simulink model "Altitude_SMCIBVS_RBFSMC"  (R2024b)
settings: Solver=FixedStepAuto  StartTime=0.0  StopTime=30  FixedStep=dT  RelTol=1e-3
InitFcn:
  | mass = 1; L = 0.2;
  | Ix = 0.008;
  | Iy = 0.008;
  | Iz = 0.017;
  | c = 0.088;
  | 
  | O = [0; 0; 0];        % world origin frame
  | C = [0; 0; 0.1];  % camera origin frame
  | 
  | d_initial = C - O;            % distance between camera and world frame
  | ang_initial = [0*pi/180  0*pi/180  0*pi/180];  % initial orientation, [pi 0 pi/2]
  | ang_final = [0*pi/180  0*pi/180  0*pi/180];
  | init_pose = [C ; ang_initial'];
  | d_final=[0; 0; 2];
  | dT=0.01;
  | g = 9.81;
  | %mass = 1; L = 0.6;
  | %Ix = 0.85;
  | %Iy = 0.85;
  | %c = 0.088;
  | 
  | p1 = [0.1; 0.1; 0.05];
  | p2 = [-0.1; 0.1; 0.05];
  | p3 = [0.1; -0.1; 0.05];
  | p4 = [-0.1; -0.1; 0.05];
  | % refcence
  | Rx = [1   0       0   ;
  |       0 cos(ang_final(1)) -sin(ang_final(1));
  |       0 sin(ang_final(1)) cos(ang_final(1))];
  | Ry = [cos(ang_final(2)) 0 sin(ang_final(2)) ;
  |        0     1   0    ;
  |      -sin(ang_final(2)) 0 cos(ang_final(2))];
  | 
  | Rz = [cos(ang_final(3)) -sin(ang_final(3)) 0;
  |       sin(ang_final(3))  cos(ang_final(3)) 0;
  |        0      0     1];
  | Rc = Rz * Ry * Rx;% body to inertial
  | Twc = [Rc            d_final;
  |       zeros(1,3)     1];
  | p_cam1 = Twc^-1 * [p1;1];   % point's position in camera frame
  | p_cam2 = Twc^-1 * [p2;1];
  | p_cam3 = Twc^-1 * [p3;1];   % point's position in camera frame
  | p_cam4 = Twc^-1 * [p4;1];
  | 
  | x_proj1 = p_cam1(1)/(p_cam1(3));%p_tilde1(1)/p_cam1(3);
  | y_proj1 = p_cam1(2)/(p_cam1(3));%p_tilde1(2)/p_cam1(3);
  | 
  | x_proj2 =p_cam2(1)/(p_cam2(3));% p_tilde2(1)/p_cam2(3);
  | y_proj2 =p_cam2(2)/(p_cam2(3));% p_tilde2(2)/p_cam2(3);
  | 
  | x_proj3 =p_cam3(1)/(p_cam3(3));% p_tilde1(1)/p_cam1(3);
  | y_proj3 =p_cam3(2)/(p_cam3(3));% p_tilde1(2)/p_cam1(3);
  | 
  | %
  | x_proj4 =p_cam4(1)/(p_cam4(3));% p_tilde2(1)/p_cam2(3);
  | y_proj4 =p_cam4(2)/(p_cam4(3));% p_tilde2(2)/p_cam2(3);
  | 
  | %%
  | ref1 = [x_proj1; y_proj1];
  | ref2 = [x_proj2; y_proj2];
  | ref3 = [x_proj3; y_proj3];
  | ref4 = [x_proj4; y_proj4];
  | 
  | ref = [ref1; ref2;ref3; ref4];
  | % control
  | %%k=[3.1383    2.9662    0.5    1.3]; %for altitude
  | k=[9.6489 9.5949 8.4692 4.5873];%for altitude new
  | 
  | kp=[k(1) k(1) k(2) k(1) k(1) k(1)];
  | kd=[k(3) k(3) k(4) k(3) k(3) k(3)];
  | %k=[1.5129    2.6987    1.6430    0.0242];%for position
  | %kp=[k(1) k(1) 5.2 k(3) k(3) 2];
  | %kd=[k(2) k(2) 4.5 k(4) k(4) 2.5];
  | 
  | Kp = diag(kp);
  | Kd = diag(kd);
  | 
  | %Rx = [1   0       0   ;
  | %      0 cos(ang_initial(1)) -sin(ang_initial(1));
  | %      0 sin(ang_initial(1)) cos(ang_initial(1))];
  | %Ry = [cos(ang_initial(2)) 0 sin(ang_initial(2)) ;
  | %       0     1   0    ;
  | %     -sin(ang_initial(2)) 0 cos(ang_initial(2))];
  | 
  | %Rz = [cos(ang_initial(3)) -sin(ang_initial(3)) 0;
  | %      sin(ang_initial(3))  cos(ang_initial(3)) 0;
  | %       0      0     1];
  | %Rc = Rz * Ry * Rx;% body to inertial
  | %Twc = [Rc            d_initial;
  | %      zeros(1,3)     1];
  | %p_cam1 = Twc^-1 * [p1;1];   % point's position in camera frame
  | %p_cam2 = Twc^-1 * [p2;1];
  | %p_cam3 = Twc^-1 * [p3;1];
  | %p_cam4 = Twc^-1 * [p4;1];
  | 
  | %x_proj1 = p_cam1(1)/(p_cam1(3));%p_tilde1(1)/p_cam1(3);
  | %y_proj1 = p_cam1(2)/(p_cam1(3));%p_tilde1(2)/p_cam1(3);
  | %Zc1 = p_cam1(3);
  | %x_proj2 =p_cam2(1)/(p_cam2(3));% p_tilde2(1)/p_cam2(3);
  | %y_proj2 =p_cam2(2)/(p_cam2(3));% p_tilde2(2)/p_cam2(3);
  | %Zc2 = p_cam2(3);
  | %x_proj3 = p_cam3(1)/(p_cam3(3));%p_tilde1(1)/p_cam1(3);
  | %y_proj3 = p_cam3(2)/(p_cam3(3));%p_tilde1(2)/p_cam1(3);
  | %Zc3 = p_cam3(3);
  | %x_proj4 =p_cam4(1)/(p_cam4(3));% p_tilde2(1)/p_cam2(3);
  | %y_proj4 =p_cam4(2)/(p_cam4(3));% p_tilde2(2)/p_cam2(3);
  | %Zc4 = p_cam4(3);
  | 
  | %ini_projection  = [x_proj1; y_proj1; Zc1; x_proj2; y_proj2; Zc2;x_proj3; y_proj3; Zc3; x_proj4; y_proj4; Zc4];
libraries: arduino_io_lib x1
settings Model: Creator=k513  LastModifiedBy=mohsen
settings DataIOCC: ReturnWorkspaceOutputs=off
settings ModelReferenceCC: EnableRefExpFcnMdlSchedulingChecks=on
settings RTWCC: GPUComputeCapability=3.5

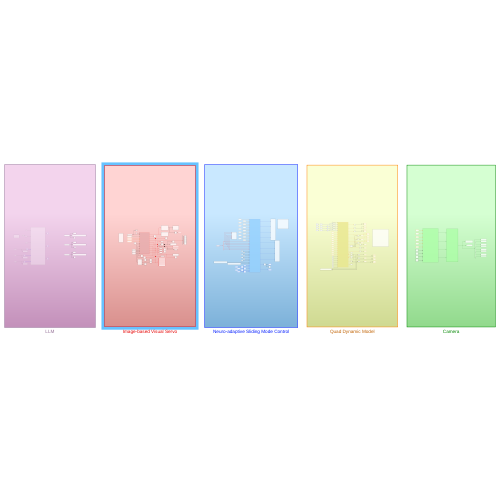
[thumbnail: Simulink's stored preview of the top-level diagram]
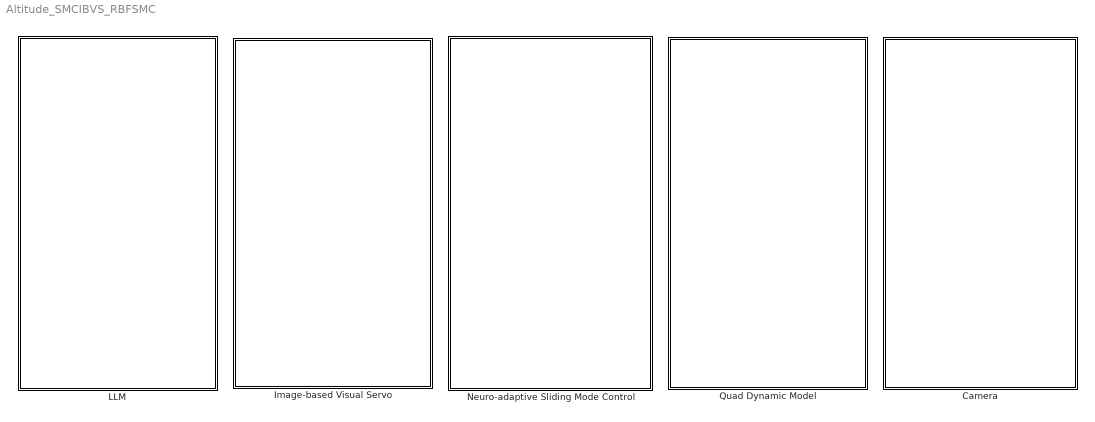
== system Altitude_SMCIBVS_RBFSMC ==
  Camera : Subsystem
  Image-based Visual Servo : Subsystem
  LLM : Subsystem
  Neuro-adaptive Sliding Mode Control : Subsystem
  Quad Dynamic Model : Subsystem

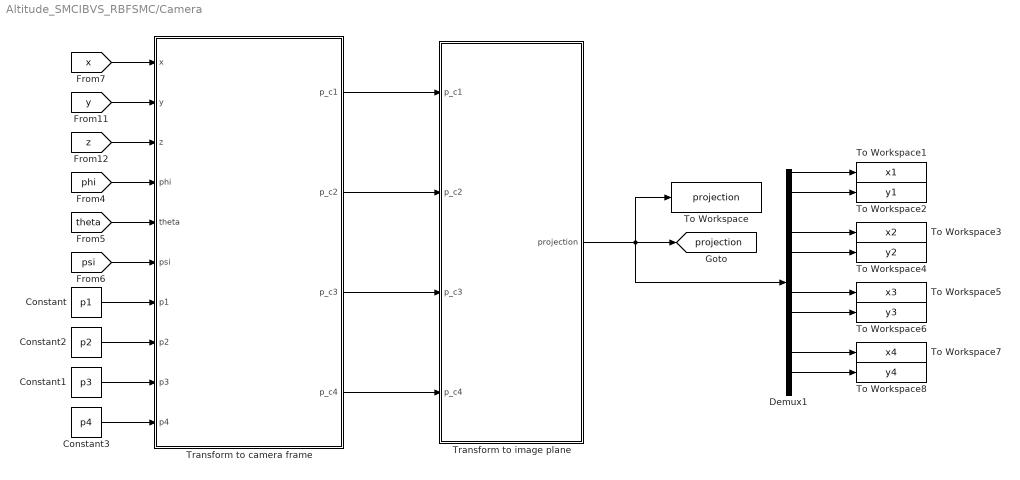
== system Altitude_SMCIBVS_RBFSMC/Camera ==
  Constant : Constant  Value=p1
  Constant1 : Constant  Value=p3
  Constant2 : Constant  Value=p2
  Constant3 : Constant  Value=p4
  Demux1 : Demux  Outputs=12
  To Workspace : ToWorkspace  VariableName=projection  SampleTime=-1
      settings: Save2DSignal=2-D array (concatenate along first dimension)
  To Workspace1 : ToWorkspace  VariableName=x1  SampleTime=-1
      settings: Save2DSignal=2-D array (concatenate along first dimension)
  To Workspace2 : ToWorkspace  VariableName=y1  SampleTime=-1
      settings: Save2DSignal=2-D array (concatenate along first dimension)
  To Workspace3 : ToWorkspace  VariableName=x2  SampleTime=-1
      settings: Save2DSignal=2-D array (concatenate along first dimension)
  To Workspace4 : ToWorkspace  VariableName=y2  SampleTime=-1
      settings: Save2DSignal=2-D array (concatenate along first dimension)
  To Workspace5 : ToWorkspace  VariableName=x3  SampleTime=-1
      settings: Save2DSignal=2-D array (concatenate along first dimension)
  To Workspace6 : ToWorkspace  VariableName=y3  SampleTime=-1
      settings: Save2DSignal=2-D array (concatenate along first dimension)
  To Workspace7 : ToWorkspace  VariableName=x4  SampleTime=-1
      settings: Save2DSignal=2-D array (concatenate along first dimension)
  To Workspace8 : ToWorkspace  VariableName=y4  SampleTime=-1
      settings: Save2DSignal=2-D array (concatenate along first dimension)
  Transform to camera frame : MATLAB Function  TreatAsAtomicUnit=on
  Transform to image plane : MATLAB Function  TreatAsAtomicUnit=on
  tag scope: projection=global
  wires:
  Transform to camera frame/1(p_c1) -> Transform to image plane/1(p_c1)
  Transform to camera frame/2(p_c2) -> Transform to image plane/2(p_c2)
  Transform to camera frame/3(p_c3) -> Transform to image plane/3(p_c3)
  Transform to camera frame/4(p_c4) -> Transform to image plane/4(p_c4)
  Demux1/2 -> To Workspace2/1
  Demux1/1 -> To Workspace1/1
  Transform to image plane/1(projection) -> To Workspace/1, Demux1/1, [projection]
  Demux1/11 -> To Workspace8/1
  Demux1/10 -> To Workspace7/1
  Demux1/8 -> To Workspace6/1
  Demux1/7 -> To Workspace5/1
  Demux1/5 -> To Workspace4/1
  Demux1/4 -> To Workspace3/1
  Constant/1 -> Transform to camera frame/7(p1)
  Constant2/1 -> Transform to camera frame/8(p2)
  Constant1/1 -> Transform to camera frame/9(p3)
  Constant3/1 -> Transform to camera frame/10(p4)
  [x] -> Transform to camera frame/1(x)
  [y] -> Transform to camera frame/2(y)
  [z] -> Transform to camera frame/3(z)
  [phi] -> Transform to camera frame/4(phi)
  [theta] -> Transform to camera frame/5(theta)
  [psi] -> Transform to camera frame/6(psi)

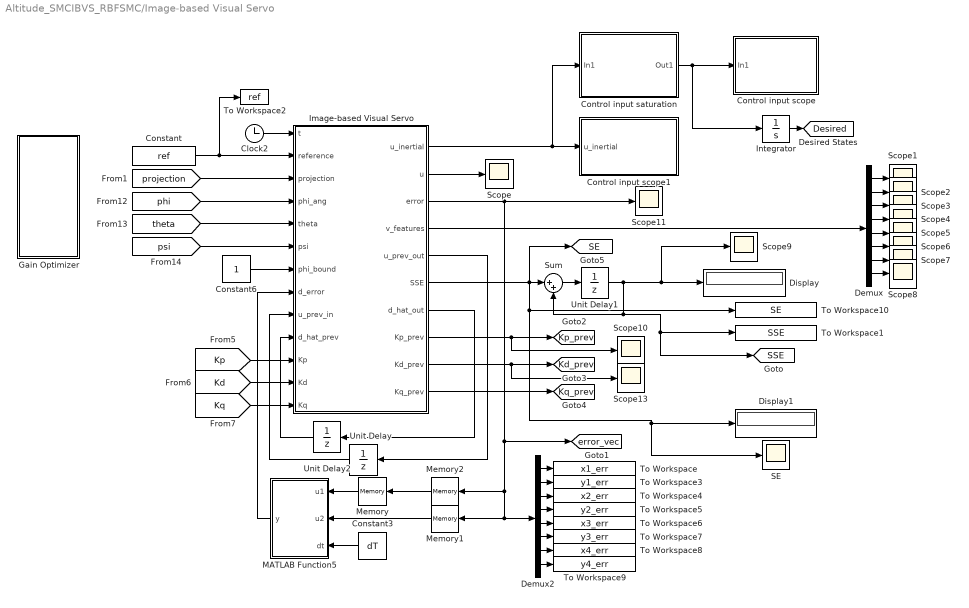
== system Altitude_SMCIBVS_RBFSMC/Image-based Visual Servo ==
  Clock2 : Clock
  Constant : Constant  Value=ref
  Constant3 : Constant  Value=dT
  Constant6 : Constant
  Control input saturation : Subsystem
  Control input scope : Subsystem
  Control input scope1 : Subsystem
  Demux : Demux  Outputs=8
  Demux2 : Demux  Outputs=8
  Display : Display
  Display1 : Display
  Gain Optimizer : Subsystem
  Image-based Visual Servo : MATLAB Function  TreatAsAtomicUnit=on
  Integrator : Integrator
  MATLAB Function5 : MATLAB Function  TreatAsAtomicUnit=on
  Memory : Memory  InitialCondition=zeros(8,1)
  Memory1 : Memory  InitialCondition=zeros(8,1)
  Memory2 : Memory  InitialCondition=zeros(8,1)
  SE : Scope
  Scope{,1..11,13} (13 alike) : Scope
  Sum : Sum  Inputs=|++
  To Workspace : ToWorkspace  VariableName=x1_err  SampleTime=-1
      settings: Save2DSignal=2-D array (concatenate along first dimension)
  To Workspace1 : ToWorkspace  VariableName=SSE  SampleTime=-1
      settings: Save2DSignal=2-D array (concatenate along first dimension)
  To Workspace10 : ToWorkspace  VariableName=SE  SampleTime=-1
      settings: Save2DSignal=2-D array (concatenate along first dimension)
  To Workspace2 : ToWorkspace  VariableName=ref  SampleTime=-1
      settings: Save2DSignal=2-D array (concatenate along first dimension)
  To Workspace3 : ToWorkspace  VariableName=y1_err  SampleTime=-1
      settings: Save2DSignal=2-D array (concatenate along first dimension)
  To Workspace4 : ToWorkspace  VariableName=x2_err  SampleTime=-1
      settings: Save2DSignal=2-D array (concatenate along first dimension)
  To Workspace5 : ToWorkspace  VariableName=y2_err  SampleTime=-1
      settings: Save2DSignal=2-D array (concatenate along first dimension)
  To Workspace6 : ToWorkspace  VariableName=x3_err  SampleTime=-1
      settings: Save2DSignal=2-D array (concatenate along first dimension)
  To Workspace7 : ToWorkspace  VariableName=y3_err  SampleTime=-1
      settings: Save2DSignal=2-D array (concatenate along first dimension)
  To Workspace8 : ToWorkspace  VariableName=x4_err  SampleTime=-1
      settings: Save2DSignal=2-D array (concatenate along first dimension)
  To Workspace9 : ToWorkspace  VariableName=y4_err  SampleTime=-1
      settings: Save2DSignal=2-D array (concatenate along first dimension)
  Unit Delay : UnitDelay  SampleTime=-1  HasFrameUpgradeWarning=on
  Unit Delay1 : UnitDelay  SampleTime=-1  HasFrameUpgradeWarning=on
  Unit Delay2 : UnitDelay  SampleTime=-1  HasFrameUpgradeWarning=on
  tag scope: Desired=global, Kd_prev=global, Kp_prev=global, Kq_prev=global, SE=global, SSE=global, error_vec=global
  wires:
  Memory/1 -> MATLAB Function5/1(u1)
  Constant/1 -> To Workspace2/1, Image-based Visual Servo/2(reference)
  [phi] -> Image-based Visual Servo/4(phi_ang)
  [theta] -> Image-based Visual Servo/5(theta)
  [psi] -> Image-based Visual Servo/6(psi)
  Image-based Visual Servo/3(error) -> Scope11/1, Demux2/1, Memory1/1, Memory2/1, [error_vec]
  [projection] -> Image-based Visual Servo/3(projection)
  Clock2/1 -> Image-based Visual Servo/1(t)
  Constant3/1 -> MATLAB Function5/3(dt)
  MATLAB Function5/1(y) -> Image-based Visual Servo/8(d_error)
  Memory1/1 -> MATLAB Function5/2(u2)
  Memory2/1 -> Memory/1
  Demux2/1 -> To Workspace/1
  Demux2/2 -> To Workspace3/1
  Demux2/3 -> To Workspace4/1
  Demux2/4 -> To Workspace5/1
  Demux2/5 -> To Workspace6/1
  Demux2/6 -> To Workspace7/1
  Demux2/7 -> To Workspace8/1
  Demux2/8 -> To Workspace9/1
  Integrator/1 -> [Desired]
  Control input saturation/1(Out1) -> Integrator/1, Control input scope/1(In1)
  Image-based Visual Servo/1(u_inertial) -> Control input saturation/1(In1), Control input scope1/1(u_inertial)
  Image-based Visual Servo/2(u) -> Scope/1
  Constant6/1 -> Image-based Visual Servo/7(phi_bound)
  Image-based Visual Servo/4(v_features) -> Demux/1
  Demux/1 -> Scope1/1
  Demux/2 -> Scope2/1
  Demux/3 -> Scope3/1
  Demux/4 -> Scope4/1
  Demux/5 -> Scope5/1
  Demux/6 -> Scope6/1
  Demux/7 -> Scope7/1
  Demux/8 -> Scope8/1
  Image-based Visual Servo/5(u_prev_out) -> Unit Delay/1
  Unit Delay/1 -> Image-based Visual Servo/9(u_prev_in)
  Image-based Visual Servo/6(SSE) -> To Workspace10/1, SE/1, Display1/1, Sum/1, [SE]
  Sum/1 -> Unit Delay1/1
  Unit Delay1/1 -> [SSE], To Workspace1/1, Sum/2, Scope9/1, Display/1
  Image-based Visual Servo/7(d_hat_out) -> Unit Delay2/1
  Unit Delay2/1 -> Image-based Visual Servo/10(d_hat_prev)
  Image-based Visual Servo/8(Kp_prev) -> Scope10/1, [Kp_prev]
  Image-based Visual Servo/9(Kd_prev) -> [Kd_prev], Scope13/1
  Image-based Visual Servo/10(Kq_prev) -> [Kq_prev]
  [Kp] -> Image-based Visual Servo/11(Kp)
  [Kd] -> Image-based Visual Servo/12(Kd)
  [Kq] -> Image-based Visual Servo/13(Kq)

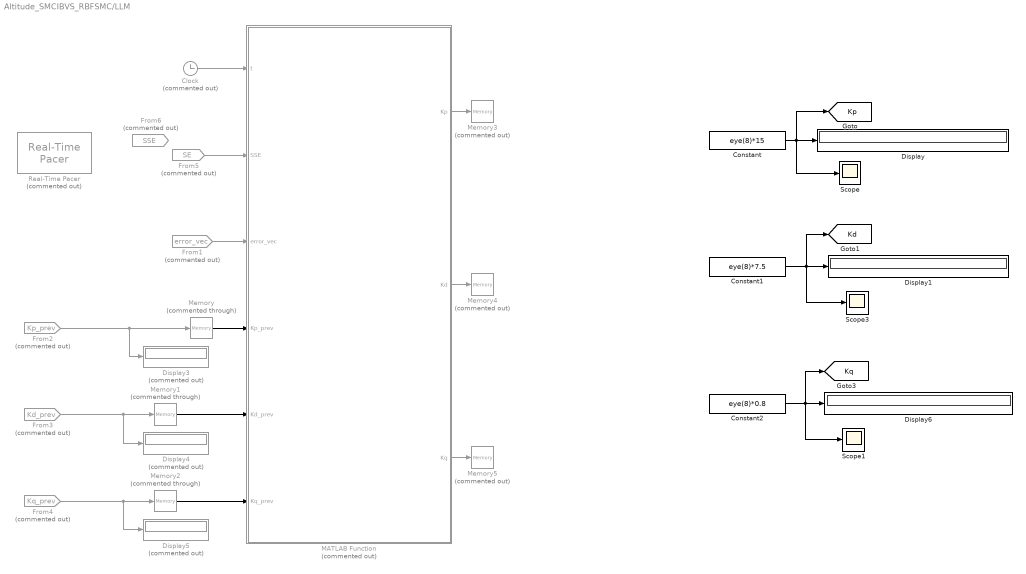
== system Altitude_SMCIBVS_RBFSMC/LLM ==
  Clock : Clock  Commented=on
  Constant : Constant  Value=eye(8)*15
  Constant1 : Constant  Value=eye(8)*7.5
  Constant2 : Constant  Value=eye(8)*0.8
  Display : Display
  Display1 : Display
  Display3 : Display  Commented=on
  Display4 : Display  Commented=on
  Display5 : Display  Commented=on
  Display6 : Display
  From1 : From  Commented=on  GotoTag=error_vec  TagVisibility=global
  From2 : From  Commented=on  GotoTag=Kp_prev  TagVisibility=global
  From3 : From  Commented=on  GotoTag=Kd_prev  TagVisibility=global
  From4 : From  Commented=on  GotoTag=Kq_prev  TagVisibility=global
  From5 : From  Commented=on  GotoTag=SE  TagVisibility=global
  From6 : From  Commented=on  GotoTag=SSE  TagVisibility=global
  MATLAB Function : MATLAB Function  Commented=on  TreatAsAtomicUnit=on
  Memory : Memory  Commented=through
  Memory1 : Memory  Commented=through
  Memory2 : Memory  Commented=through
  Memory3 : Memory  Commented=on
  Memory4 : Memory  Commented=on
  Memory5 : Memory  Commented=on
  Real-Time Pacer : arduino_io_lib/Real-Time Pacer  Commented=on  simTimePerRealTime=1
      settings: SourceProductName=Arduino IO Library
  Scope : Scope
  Scope1 : Scope
  Scope3 : Scope
  tag scope: Kd=global, Kp=global, Kq=global
  wires:
  MATLAB Function/1(Kp) -> Memory3/1
  MATLAB Function/3(Kq) -> Memory5/1
  MATLAB Function/2(Kd) -> Memory4/1
  Clock/1 -> MATLAB Function/1(t)
  From1/1 -> MATLAB Function/3(error_vec)
  From5/1 -> MATLAB Function/2(SSE)
  Memory/1 -> MATLAB Function/4(Kp_prev)
  Memory1/1 -> MATLAB Function/5(Kd_prev)
  Memory2/1 -> MATLAB Function/6(Kq_prev)
  From2/1 -> Display3/1, Memory/1
  From3/1 -> Display4/1, Memory1/1
  From4/1 -> Memory2/1, Display5/1
  Constant/1 -> Scope/1, [Kp], Display/1
  Constant1/1 -> Scope3/1, [Kd], Display1/1
  Constant2/1 -> Scope1/1, Display6/1, [Kq]

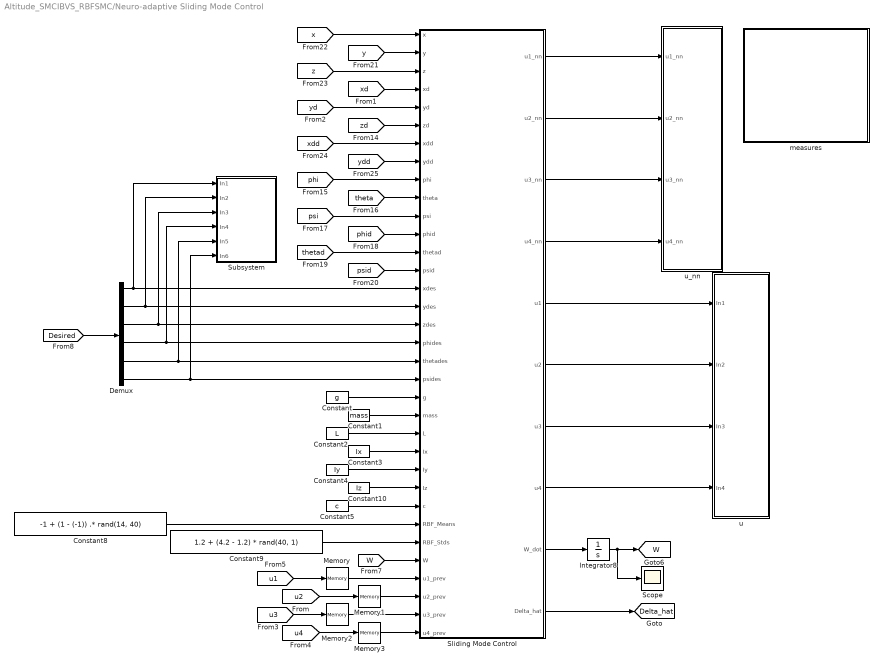
== system Altitude_SMCIBVS_RBFSMC/Neuro-adaptive Sliding Mode Control ==
  Constant : Constant  Value=g
  Constant1 : Constant  Value=mass
  Constant10 : Constant  Value=Iz
  Constant2 : Constant  Value=L
  Constant3 : Constant  Value=Ix
  Constant4 : Constant  Value=Iy
  Constant5 : Constant  Value=c
  Constant8 : Constant  Value=-1 + (1 - (-1)) .* rand(14, 40)
  Constant9 : Constant  Value=1.2 + (4.2 - 1.2) * rand(40, 1)
  Demux : Demux  Outputs=6
  Integrator8 : Integrator  InitialCondition=zeros(40, 4)
  Memory{,1..3} (4 alike) : Memory
  Scope : Scope
  Sliding Mode Control : MATLAB Function  TreatAsAtomicUnit=on
  Subsystem : Subsystem
  measures : Subsystem
  u : Subsystem
  u_nn : Subsystem
  tag scope: Delta_hat=global, W=global
  wires:
  [theta] -> Sliding Mode Control/10(theta)
  [zd] -> Sliding Mode Control/6(zd)
  [yd] -> Sliding Mode Control/5(yd)
  [xdd] -> Sliding Mode Control/7(xdd)
  [thetad] -> Sliding Mode Control/13(thetad)
  [phid] -> Sliding Mode Control/12(phid)
  [psi] -> Sliding Mode Control/11(psi)
  [ydd] -> Sliding Mode Control/8(ydd)
  [y] -> Sliding Mode Control/2(y)
  [phi] -> Sliding Mode Control/9(phi)
  [xd] -> Sliding Mode Control/4(xd)
  [psid] -> Sliding Mode Control/14(psid)
  [x] -> Sliding Mode Control/1(x)
  [z] -> Sliding Mode Control/3(z)
  [Desired] -> Demux/1
  Demux/3 -> Subsystem/3(In3), Sliding Mode Control/17(zdes)
  Constant/1 -> Sliding Mode Control/21(g)
  Constant1/1 -> Sliding Mode Control/22(mass)
  Constant2/1 -> Sliding Mode Control/23(L)
  Constant3/1 -> Sliding Mode Control/24(Ix)
  Constant4/1 -> Sliding Mode Control/25(Iy)
  Constant5/1 -> Sliding Mode Control/27(c)
  Constant10/1 -> Sliding Mode Control/26(Iz)
  Constant9/1 -> Sliding Mode Control/29(RBF_Stds)
  Constant8/1 -> Sliding Mode Control/28(RBF_Means)
  Sliding Mode Control/9(W_dot) -> Integrator8/1
  [u1] -> Memory/1
  [u2] -> Memory1/1
  [u3] -> Memory2/1
  [u4] -> Memory3/1
  Memory/1 -> Sliding Mode Control/31(u1_prev)
  Memory1/1 -> Sliding Mode Control/32(u2_prev)
  Memory2/1 -> Sliding Mode Control/33(u3_prev)
  Memory3/1 -> Sliding Mode Control/34(u4_prev)
  Sliding Mode Control/10(Delta_hat) -> [Delta_hat]
  Integrator8/1 -> Scope/1, [W]
  [W] -> Sliding Mode Control/30(W)
  Demux/1 -> Subsystem/1(In1), Sliding Mode Control/15(xdes)
  Demux/2 -> Subsystem/2(In2), Sliding Mode Control/16(ydes)
  Demux/4 -> Subsystem/4(In4), Sliding Mode Control/18(phides)
  Demux/5 -> Subsystem/5(In5), Sliding Mode Control/19(thetades)
  Demux/6 -> Subsystem/6(In6), Sliding Mode Control/20(psides)
  Sliding Mode Control/1(u1_nn) -> u_nn/1(u1_nn)
  Sliding Mode Control/2(u2_nn) -> u_nn/2(u2_nn)
  Sliding Mode Control/3(u3_nn) -> u_nn/3(u3_nn)
  Sliding Mode Control/4(u4_nn) -> u_nn/4(u4_nn)
  Sliding Mode Control/5(u1) -> u/1(In1)
  Sliding Mode Control/6(u2) -> u/2(In2)
  Sliding Mode Control/7(u3) -> u/3(In3)
  Sliding Mode Control/8(u4) -> u/4(In4)

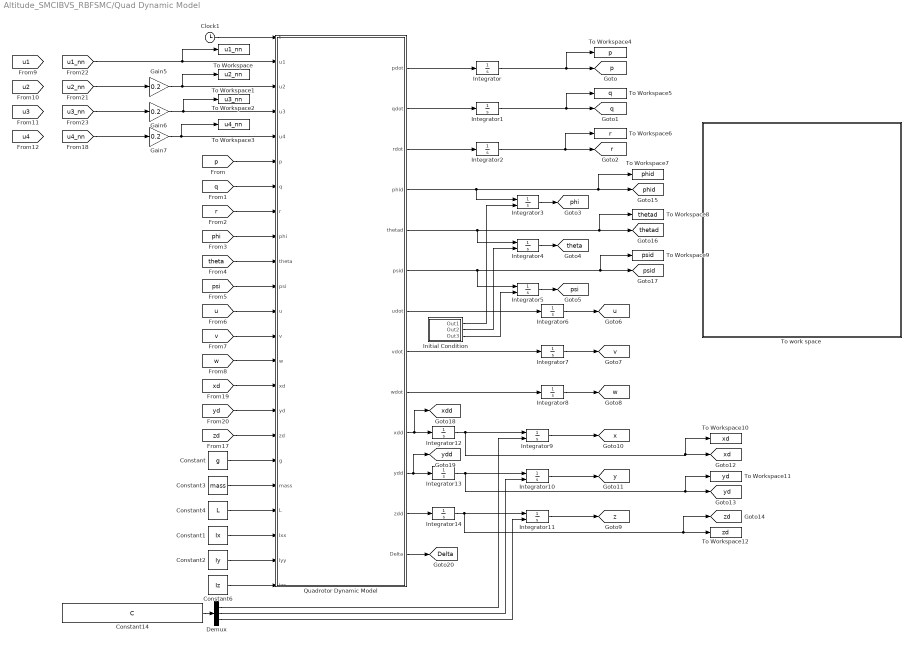
== system Altitude_SMCIBVS_RBFSMC/Quad Dynamic Model ==
  Clock1 : Clock
  Constant : Constant  Value=g
  Constant1 : Constant  Value=Ix
  Constant14 : Constant  Value=C
  Constant2 : Constant  Value=Iy
  Constant3 : Constant  Value=mass
  Constant4 : Constant  Value=L
  Constant6 : Constant  Value=Iz
  Demux : Demux  Outputs=3
  Gain5 : Gain  Gain=0.2
  Gain6 : Gain  Gain=0.2
  Gain7 : Gain  Gain=0.2
  Initial Condition : Subsystem
  Integrator : Integrator  InitialCondition=-0.003775510005653
  Integrator1 : Integrator  InitialCondition=0.003931066952646
  Integrator{3..5,9..11} (6 alike) : Integrator  InitialConditionSource=external
  Integrator{6..8,12..14} (6 alike) : Integrator
  Integrator2 : Integrator  InitialCondition=0.005723309703171
  Quadrotor Dynamic Model : MATLAB Function  TreatAsAtomicUnit=on
  To Workspace : ToWorkspace  VariableName=u1_nn  SampleTime=-1
      settings: Save2DSignal=2-D array (concatenate along first dimension)
  To Workspace1 : ToWorkspace  VariableName=u2_nn  SampleTime=-1
      settings: Save2DSignal=2-D array (concatenate along first dimension)
  To Workspace10 : ToWorkspace  VariableName=xd  SampleTime=-1
  To Workspace11 : ToWorkspace  VariableName=yd  SampleTime=-1
  To Workspace12 : ToWorkspace  VariableName=zd  SampleTime=-1
  To Workspace2 : ToWorkspace  VariableName=u3_nn  SampleTime=-1
      settings: Save2DSignal=2-D array (concatenate along first dimension)
  To Workspace3 : ToWorkspace  VariableName=u4_nn  SampleTime=-1
      settings: Save2DSignal=2-D array (concatenate along first dimension)
  To Workspace4 : ToWorkspace  VariableName=p  SampleTime=-1
  To Workspace5 : ToWorkspace  VariableName=q  SampleTime=-1
  To Workspace6 : ToWorkspace  VariableName=r  SampleTime=-1
  To Workspace7 : ToWorkspace  VariableName=phid  SampleTime=-1
  To Workspace8 : ToWorkspace  VariableName=thetad  SampleTime=-1
  To Workspace9 : ToWorkspace  VariableName=psid  SampleTime=-1
  To work space : Subsystem
  tag scope: Delta=global, p=global, phi=global, phid=global, psi=global, psid=global, q=global, r=global, theta=global, thetad=global, u=global, v=global, w=global, x=global, xd=global, xdd=global, y=global, yd=global, ydd=global, z=global, zd=global
  wires:
  [theta] -> Quadrotor Dynamic Model/10(theta)
  [psi] -> Quadrotor Dynamic Model/11(psi)
  Constant14/1 -> Demux/1
  Quadrotor Dynamic Model/11(ydd) -> Integrator13/1, [ydd]
  Quadrotor Dynamic Model/2(qdot) -> Integrator1/1
  Constant6/1 -> Quadrotor Dynamic Model/23(Izz)
  [r] -> Quadrotor Dynamic Model/8(r)
  Quadrotor Dynamic Model/3(rdot) -> Integrator2/1
  Integrator/1 -> To Workspace4/1, [p]
  Quadrotor Dynamic Model/13(Delta) -> [Delta]
  Integrator2/1 -> To Workspace6/1, [r]
  Quadrotor Dynamic Model/5(thetad) -> Integrator4/1, [thetad], To Workspace8/1
  [q] -> Quadrotor Dynamic Model/7(q)
  Quadrotor Dynamic Model/4(phid) -> Integrator3/1, [phid], To Workspace7/1
  [yd] -> Quadrotor Dynamic Model/16(yd)
  Demux/2 -> Integrator10/2
  Demux/3 -> Integrator11/2
  Integrator12/1 -> [xd], To Workspace10/1, Integrator9/1
  Quadrotor Dynamic Model/8(vdot) -> Integrator7/1
  Integrator4/1 -> [theta]
  Integrator6/1 -> [u]
  Integrator13/1 -> [yd], To Workspace11/1, Integrator10/1
  Integrator11/1 -> [z]
  Integrator1/1 -> To Workspace5/1, [q]
  Quadrotor Dynamic Model/12(zdd) -> Integrator14/1
  Quadrotor Dynamic Model/9(wdot) -> Integrator8/1
  Integrator5/1 -> [psi]
  Demux/1 -> Integrator9/2
  [xd] -> Quadrotor Dynamic Model/15(xd)
  [u] -> Quadrotor Dynamic Model/12(u)
  [phi] -> Quadrotor Dynamic Model/9(phi)
  Gain7/1 -> Quadrotor Dynamic Model/5(u4), To Workspace3/1
  Integrator7/1 -> [v]
  Integrator3/1 -> [phi]
  Constant1/1 -> Quadrotor Dynamic Model/21(Ixx)
  Integrator14/1 -> [zd], To Workspace12/1, Integrator11/1
  Gain5/1 -> To Workspace1/1, Quadrotor Dynamic Model/3(u2)
  [p] -> Quadrotor Dynamic Model/6(p)
  Constant3/1 -> Quadrotor Dynamic Model/19(mass)
  Integrator8/1 -> [w]
  Quadrotor Dynamic Model/6(psid) -> To Workspace9/1, [psid], Integrator5/1
  Integrator9/1 -> [x]
  Quadrotor Dynamic Model/10(xdd) -> Integrator12/1, [xdd]
  [v] -> Quadrotor Dynamic Model/13(v)
  Gain6/1 -> To Workspace2/1, Quadrotor Dynamic Model/4(u3)
  [w] -> Quadrotor Dynamic Model/14(w)
  Constant2/1 -> Quadrotor Dynamic Model/22(Iyy)
  [zd] -> Quadrotor Dynamic Model/17(zd)
  Quadrotor Dynamic Model/7(udot) -> Integrator6/1
  Integrator10/1 -> [y]
  Clock1/1 -> Quadrotor Dynamic Model/1(t)
  Constant4/1 -> Quadrotor Dynamic Model/20(L)
  Quadrotor Dynamic Model/1(pdot) -> Integrator/1
  Constant/1 -> Quadrotor Dynamic Model/18(g)
  Initial Condition/1(Out1) -> Integrator3/2
  Initial Condition/2(Out2) -> Integrator4/2
  Initial Condition/3(Out3) -> Integrator5/2
  [u1_nn] -> To Workspace/1, Quadrotor Dynamic Model/2(u1)
  [u2_nn] -> Gain5/1
  [u3_nn] -> Gain6/1
  [u4_nn] -> Gain7/1

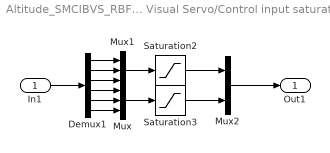
== system Altitude_SMCIBVS_RBFSMC/Image-based Visual Servo/Control input saturation ==
  In1 : Inport
  Demux1 : Demux  Outputs=6
  Mux : Mux  Inputs=3
  Mux1 : Mux  Inputs=3
  Mux2 : Mux  Inputs=2
  Saturation2 : Saturate  UpperLimit=1  LowerLimit=-1
  Saturation3 : Saturate
  Out1 : Outport
  wires:
  Mux1/1 -> Saturation2/1
  Demux1/3 -> Mux1/3
  Saturation2/1 -> Mux2/1
  Demux1/4 -> Mux/1
  Demux1/2 -> Mux1/2
  Demux1/5 -> Mux/2
  Demux1/6 -> Mux/3
  Demux1/1 -> Mux1/1
  Saturation3/1 -> Mux2/2
  Mux/1 -> Saturation3/1
  In1/1 -> Demux1/1
  Mux2/1 -> Out1/1

== system Altitude_SMCIBVS_RBFSMC/Image-based Visual Servo/Control input scope ==
  In1 : Inport
  Demux : Demux  Outputs=6
  Scope1 : Scope  NumInputPorts=3
  Scope2 : Scope  NumInputPorts=3
  wires:
  Demux/2 -> Scope1/2
  Demux/4 -> Scope2/1
  Demux/6 -> Scope2/3
  Demux/1 -> Scope1/1
  Demux/3 -> Scope1/3
  In1/1 -> Demux/1
  Demux/5 -> Scope2/2

== system Altitude_SMCIBVS_RBFSMC/Image-based Visual Servo/Control input scope1 ==
  u_inertial : Inport
  Demux : Demux  Outputs=6
  Scope1 : Scope  NumInputPorts=3
  Scope2 : Scope  NumInputPorts=3
  wires:
  Demux/5 -> Scope2/2
  u_inertial/1 -> Demux/1
  Demux/3 -> Scope1/3
  Demux/1 -> Scope1/1
  Demux/6 -> Scope2/3
  Demux/4 -> Scope2/1
  Demux/2 -> Scope1/2

== system Altitude_SMCIBVS_RBFSMC/Image-based Visual Servo/Gain Optimizer ==
  Abs : Abs  SaturateOnIntegerOverflow=off
  Clock : Clock
  Display1 : Display
  Integrator : Integrator
  MATLAB Function : MATLAB Function  TreatAsAtomicUnit=on
  Product : Product
  To Workspace1 : ToWorkspace  VariableName=ITAE  SampleTime=-1
      settings: Save2DSignal=2-D array (concatenate along first dimension)
  wires:
  Integrator/1 -> Product/1
  Product/1 -> To Workspace1/1, Display1/1
  MATLAB Function/1(y) -> Abs/1
  [error] -> MATLAB Function/1(u)
  Abs/1 -> Integrator/1
  Clock/1 -> Product/2

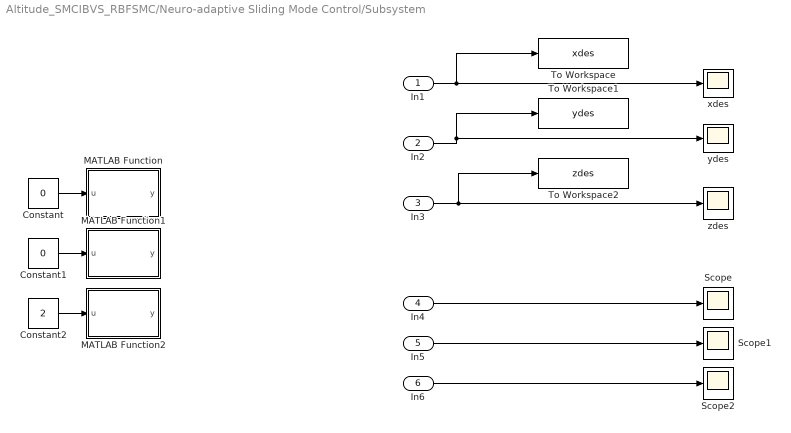
== system Altitude_SMCIBVS_RBFSMC/Neuro-adaptive Sliding Mode Control/Subsystem ==
  In1 : Inport
  In2 : Inport  Port=2
  In3 : Inport  Port=3
  In4 : Inport  Port=4
  In5 : Inport  Port=5
  In6 : Inport  Port=6
  Constant : Constant  Value=0
  Constant1 : Constant  Value=0
  Constant2 : Constant  Value=2
  MATLAB Function : MATLAB Function  TreatAsAtomicUnit=on
  MATLAB Function1 : MATLAB Function  TreatAsAtomicUnit=on
  MATLAB Function2 : MATLAB Function  TreatAsAtomicUnit=on
  Scope : Scope
  Scope1 : Scope
  Scope2 : Scope
  To Workspace : ToWorkspace  VariableName=xdes  SampleTime=-1
      settings: Save2DSignal=2-D array (concatenate along first dimension)
  To Workspace1 : ToWorkspace  VariableName=ydes  SampleTime=-1
      settings: Save2DSignal=2-D array (concatenate along first dimension)
  To Workspace2 : ToWorkspace  VariableName=zdes  SampleTime=-1
      settings: Save2DSignal=2-D array (concatenate along first dimension)
  xdes : Scope
  ydes : Scope
  zdes : Scope
  wires:
  In2/1 -> ydes/1, To Workspace1/1
  In3/1 -> To Workspace2/1, zdes/1
  In1/1 -> To Workspace/1, xdes/1
  In4/1 -> Scope/1
  In5/1 -> Scope1/1
  In6/1 -> Scope2/1
  Constant/1 -> MATLAB Function/1(u)
  Constant1/1 -> MATLAB Function1/1(u)
  Constant2/1 -> MATLAB Function2/1(u)

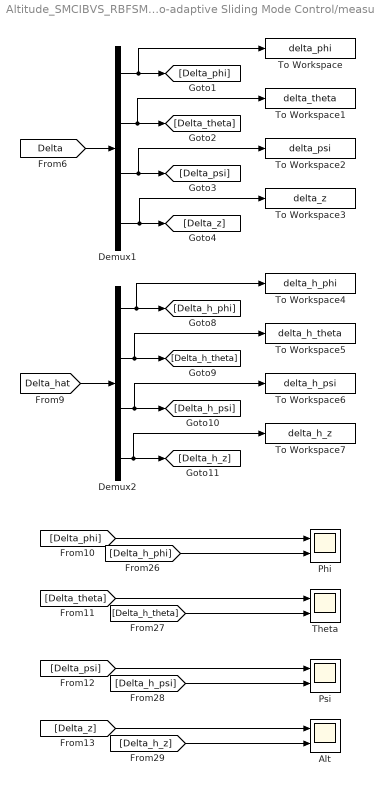
== system Altitude_SMCIBVS_RBFSMC/Neuro-adaptive Sliding Mode Control/measures ==
  Alt : Scope  NumInputPorts=2
  Demux1 : Demux
  Demux2 : Demux
  Phi : Scope  NumInputPorts=2
  Psi : Scope  NumInputPorts=2
  Theta : Scope  NumInputPorts=2
  To Workspace : ToWorkspace  VariableName=delta_phi  SampleTime=-1
      settings: Save2DSignal=2-D array (concatenate along first dimension)
  To Workspace1 : ToWorkspace  VariableName=delta_theta  SampleTime=-1
      settings: Save2DSignal=2-D array (concatenate along first dimension)
  To Workspace2 : ToWorkspace  VariableName=delta_psi  SampleTime=-1
      settings: Save2DSignal=2-D array (concatenate along first dimension)
  To Workspace3 : ToWorkspace  VariableName=delta_z  SampleTime=-1
      settings: Save2DSignal=2-D array (concatenate along first dimension)
  To Workspace4 : ToWorkspace  VariableName=delta_h_phi  SampleTime=-1
      settings: Save2DSignal=2-D array (concatenate along first dimension)
  To Workspace5 : ToWorkspace  VariableName=delta_h_theta  SampleTime=-1
      settings: Save2DSignal=2-D array (concatenate along first dimension)
  To Workspace6 : ToWorkspace  VariableName=delta_h_psi  SampleTime=-1
      settings: Save2DSignal=2-D array (concatenate along first dimension)
  To Workspace7 : ToWorkspace  VariableName=delta_h_z  SampleTime=-1
      settings: Save2DSignal=2-D array (concatenate along first dimension)
  wires:
  [Delta_h_phi] -> Phi/2
  Demux1/1 -> To Workspace/1, [Delta_phi]
  [Delta_h_theta] -> Theta/2
  [Delta] -> Demux1/1
  Demux2/2 -> To Workspace5/1, [Delta_h_theta]
  [Delta_hat] -> Demux2/1
  Demux1/3 -> To Workspace2/1, [Delta_psi]
  Demux2/4 -> To Workspace7/1, [Delta_h_z]
  [Delta_psi] -> Psi/1
  Demux2/3 -> To Workspace6/1, [Delta_h_psi]
  [Delta_h_psi] -> Psi/2
  Demux1/4 -> To Workspace3/1, [Delta_z]
  Demux1/2 -> To Workspace1/1, [Delta_theta]
  [Delta_h_z] -> Alt/2
  [Delta_theta] -> Theta/1
  [Delta_phi] -> Phi/1
  [Delta_z] -> Alt/1
  Demux2/1 -> To Workspace4/1, [Delta_h_phi]

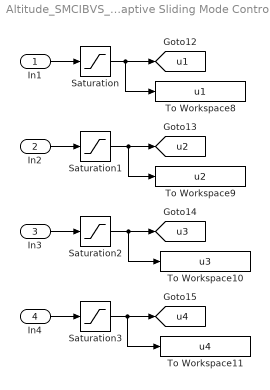
== system Altitude_SMCIBVS_RBFSMC/Neuro-adaptive Sliding Mode Control/u ==
  In1 : Inport
  In2 : Inport  Port=2
  In3 : Inport  Port=3
  In4 : Inport  Port=4
  Saturation : Saturate  UpperLimit=400  LowerLimit=-350
  Saturation1 : Saturate  UpperLimit=8  LowerLimit=-8
  Saturation2 : Saturate  UpperLimit=8  LowerLimit=-8
  Saturation3 : Saturate  UpperLimit=4  LowerLimit=-3
  To Workspace10 : ToWorkspace  VariableName=u3  SampleTime=-1
      settings: Save2DSignal=2-D array (concatenate along first dimension)
  To Workspace11 : ToWorkspace  VariableName=u4  SampleTime=-1
      settings: Save2DSignal=2-D array (concatenate along first dimension)
  To Workspace8 : ToWorkspace  VariableName=u1  SampleTime=-1
      settings: Save2DSignal=2-D array (concatenate along first dimension)
  To Workspace9 : ToWorkspace  VariableName=u2  SampleTime=-1
      settings: Save2DSignal=2-D array (concatenate along first dimension)
  tag scope: u1=global, u2=global, u3=global, u4=global
  wires:
  In4/1 -> Saturation3/1
  Saturation1/1 -> To Workspace9/1, [u2]
  Saturation2/1 -> To Workspace10/1, [u3]
  Saturation3/1 -> To Workspace11/1, [u4]
  In1/1 -> Saturation/1
  In3/1 -> Saturation2/1
  Saturation/1 -> To Workspace8/1, [u1]
  In2/1 -> Saturation1/1

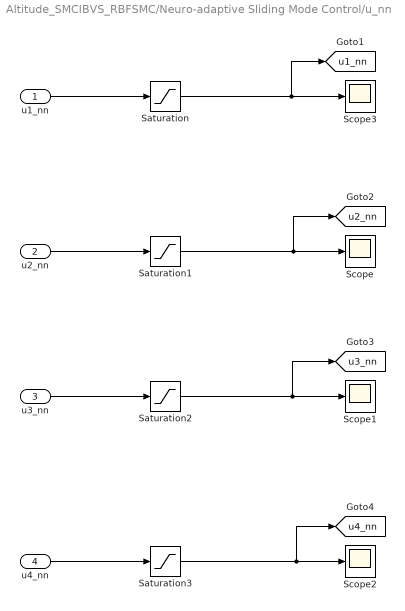
== system Altitude_SMCIBVS_RBFSMC/Neuro-adaptive Sliding Mode Control/u_nn ==
  u1_nn : Inport
  u2_nn : Inport  Port=2
  u3_nn : Inport  Port=3
  u4_nn : Inport  Port=4
  Saturation : Saturate  UpperLimit=400  LowerLimit=-350
  Saturation1 : Saturate  UpperLimit=8  LowerLimit=-8
  Saturation2 : Saturate  UpperLimit=8  LowerLimit=-8
  Saturation3 : Saturate  UpperLimit=4  LowerLimit=-3
  Scope{,1..3} (4 alike) : Scope
  tag scope: u1_nn=global, u2_nn=global, u3_nn=global, u4_nn=global
  wires:
  Saturation/1 -> Scope3/1, [u1_nn]
  u4_nn/1 -> Saturation3/1
  Saturation2/1 -> [u3_nn], Scope1/1
  u3_nn/1 -> Saturation2/1
  Saturation3/1 -> [u4_nn], Scope2/1
  u2_nn/1 -> Saturation1/1
  Saturation1/1 -> Scope/1, [u2_nn]
  u1_nn/1 -> Saturation/1

== system Altitude_SMCIBVS_RBFSMC/Quad Dynamic Model/Initial Condition ==
  Constant5 : Constant  Value=ang_initial
  Demux1 : Demux  Outputs=3
  Out1 : Outport
  Out2 : Outport  Port=2
  Out3 : Outport  Port=3
  wires:
  Constant5/1 -> Demux1/1
  Demux1/2 -> Out2/1
  Demux1/1 -> Out1/1
  Demux1/3 -> Out3/1

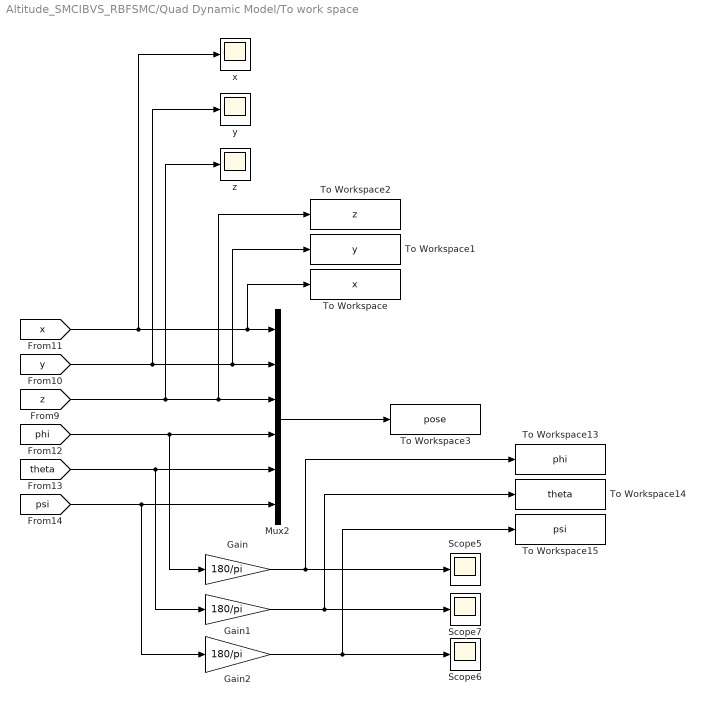
== system Altitude_SMCIBVS_RBFSMC/Quad Dynamic Model/To work space ==
  Gain : Gain  Gain=180/pi
  Gain1 : Gain  Gain=180/pi
  Gain2 : Gain  Gain=180/pi
  Mux2 : Mux  Inputs=6
  Scope5 : Scope
  Scope6 : Scope
  Scope7 : Scope
  To Workspace : ToWorkspace  VariableName=x  SampleTime=-1
      settings: Save2DSignal=2-D array (concatenate along first dimension)
  To Workspace1 : ToWorkspace  VariableName=y  SampleTime=-1
      settings: Save2DSignal=2-D array (concatenate along first dimension)
  To Workspace13 : ToWorkspace  VariableName=phi  SampleTime=-1
      settings: Save2DSignal=2-D array (concatenate along first dimension)
  To Workspace14 : ToWorkspace  VariableName=theta  SampleTime=-1
      settings: Save2DSignal=2-D array (concatenate along first dimension)
  To Workspace15 : ToWorkspace  VariableName=psi  SampleTime=-1
      settings: Save2DSignal=2-D array (concatenate along first dimension)
  To Workspace2 : ToWorkspace  VariableName=z  SampleTime=-1
      settings: Save2DSignal=2-D array (concatenate along first dimension)
  To Workspace3 : ToWorkspace  VariableName=pose  SampleTime=-1
      settings: Save2DSignal=2-D array (concatenate along first dimension)
  x : Scope
  y : Scope
  z : Scope
  wires:
  [theta] -> Gain1/1, Mux2/5
  Gain2/1 -> Scope6/1, To Workspace15/1
  Gain1/1 -> Scope7/1, To Workspace14/1
  [x] -> Mux2/1, To Workspace/1, x/1
  [y] -> Mux2/2, To Workspace1/1, y/1
  [z] -> Mux2/3, To Workspace2/1, z/1
  [psi] -> Mux2/6, Gain2/1
  [phi] -> Gain/1, Mux2/4
  Gain/1 -> Scope5/1, To Workspace13/1
  Mux2/1 -> To Workspace3/1

== matlab function Altitude_SMCIBVS_RBFSMC/LLM/MATLAB Function ==
  settings: updateMethod=DISCRETE  sampleTime=0.01
  data: t input; SSE input; Kp output; error_vec input; Kp_prev input; Kd_prev input; Kq_prev input; Kd output; Kq output
function [Kp, Kd, Kq] = LLM_Agent_Bridge(t, SSE, error_vec, Kp_prev, Kd_prev, Kq_prev)
   
    Kp = zeros(8,8); Kd = zeros(8,8); Kq = zeros(8,8);
    
    persistent t0 Kp_p Kd_p Kq_p 
    if isempty(t0)
        t0 = 0;
        % Kp_p = eye(8)*15; 
        % Kd_p = eye(8)*7.5; 
        % Kq_p = eye(8)*0.8;
        % Kp_p = eye(8)*17;
        % Kd_p = eye(8)*8;
        % Kq_p = eye(8)*0.85;

        Kp_p = eye(8)*18;
        Kd_p = eye(8)*8.2;
        Kq_p = eye(8)*0.9;


    end
    % if t < 5
    %     Kp = eye(8)*15; Kd = eye(8)*7.5; Kq = eye(8)*0.8;
    % end

    if (t - t0) >= 15.0

        tel.SSE = SSE;
        tel.max_err = max(abs(error_vec));
        tel.Kp = Kp_p(1,1);

        save('telemetry.mat', 'tel');

        if exist('gains_from_llm.mat', 'file')
            S = load('gains_from_llm.mat');
            coder.varsize('S.new_gains.reason', [1 100], [false false]);
            if isfield(S, 'new_gains')
                prop = S.new_gains;

                prop.Kp = max(10, min(20, prop.Kp));
                % prop.Kp = 15;
                

                prop.Kd = max(4.5, min(11.5, prop.Kd));
                % prop.Kd = 7.5;
                

                prop.Kq = max(0.5, min(1.2, prop.Kq));
                % prop.Kq = 0.8;
                
                Kp_p = eye(8) * prop.Kp;
                Kd_p = eye(8) * prop.Kd;
                Kq_p = eye(8) * prop.Kq;
            end
        end
        t0 = t;
    end

    Kp = Kp_p; Kd = Kd_p; Kq = Kq_p;
end

== matlab function Altitude_SMCIBVS_RBFSMC/Camera/Transform to image plane ==
  data: p_c1 input; p_c2 input; p_c3 input; p_c4 input; projection output size=12
function projection = project_to_image_plane(p_c1, p_c2, p_c3, p_c4)

x_i1 = p_c1(1)/p_c1(3);
y_i1 = p_c1(2)/p_c1(3);
z_c1 = p_c1(3);

x_i2 = p_c2(1)/p_c2(3);
y_i2 = p_c2(2)/p_c2(3);
z_c2 = p_c2(3);

x_i3 = p_c3(1)/p_c3(3);
y_i3 = p_c3(2)/p_c3(3);
z_c3 = p_c3(3);

x_i4 = p_c4(1)/p_c4(3);
y_i4 = p_c4(2)/p_c4(3);
z_c4 = p_c4(3);


projection  = [x_i1; y_i1; z_c1; x_i2; y_i2; z_c2; x_i3; y_i3; z_c3; x_i4; y_i4; z_c4];

== matlab function Altitude_SMCIBVS_RBFSMC/Camera/Transform to camera frame ==
  data: x input; p_c1 output; y input; z input; phi input; theta input; psi input; p_c2 output; p_c3 output; p_c4 output; p1 input; p2 input; p3 input; p4 input
%function [xc, yc, zc] = transform_to_camera_frame(x, y, z, phi, theta, psi)
function [p_c1, p_c2, p_c3, p_c4] = transform_to_camera_frame(x, y, z, phi, theta, psi,p1,p2,p3,p4)

    d = [x; y; z];
    % % points' position (x,y,z) in world frame

    % Define rotation matrices for each Euler angle
    Rx = [1 0 0; 0 cos(phi) -sin(phi); 0 sin(phi) cos(phi)];
    Ry = [cos(theta) 0 sin(theta); 0 1 0; -sin(theta) 0 cos(theta)];
    Rz = [cos(psi) -sin(psi) 0; sin(psi) cos(psi) 0; 0 0 1];
    
    % Compute the combined rotation matrix
    R = Rz * Ry * Rx;

    % Twc = [R            d;
    %       zeros(1,3)     1];
    Twc = [R d; 0 0 0 1];
    
    
    p_c1 = Twc \ [p1; 1];   % point's position in camera frame
    p_c2 = Twc \ [p2; 1];
    p_c3 = Twc \ [p3; 1];   
    p_c4 = Twc \ [p4; 1];
end       
%     % Transform the position to the camera frame
%     position_global = [x; y; z];
%     position_camera = R * position_global;
%     
%     % Extract x, y, and z components in the camera frame
%     xc = position_camera(1);
%     yc = position_camera(2);
%     zc = position_camera(3);

== matlab function Altitude_SMCIBVS_RBFSMC/Neuro-adaptive Sliding Mode Control/Subsystem/MATLAB Function ==
  data: u input; y output
function y = fcn(u)

y = u;

== matlab function Altitude_SMCIBVS_RBFSMC/Neuro-adaptive Sliding Mode Control/Sliding Mode Control ==
  data: u1_nn output; u2_nn output; u3_nn output; u4_nn output; u1 output; x input; y input; z input; xd input; yd input; zd input; xdd input; ydd input; phi input; theta input; psi input; phid input; thetad input; psid input; xdes input; ydes input; zdes input; phides input; thetades input; u2 output; u3 output; u4 output; psides input; g input; mass input; L input; Ix input; Iy input; Iz input; c input; RBF_Means input; RBF_Stds input; W_dot output; W input; u1_prev input; u2_prev input; u3_prev input; u4_prev input; Delta_hat output
function [u1_nn, u2_nn, u3_nn, u4_nn, u1, u2, u3, u4, W_dot, Delta_hat] = fcn(x, y, z, xd, yd, zd, xdd, ydd, phi, theta, psi, phid, thetad, psid, xdes, ydes, zdes, phides, thetades, psides, g, mass, L, Ix, Iy, Iz, c, RBF_Means, RBF_Stds, W, u1_prev, u2_prev, u3_prev, u4_prev)
% nfunction [u1_nn, u2_nn, u3_nn, u4_nn, u1, u2, u3, u4, W_dot, Delta_hat]     = fcn(x,y,z,xd,yd,zd,xdd,ydd,phi,theta,psi,phid,thetad,psid, xdes, ydes, zdes,phides, thetades,psides,g,mass,L,Ix,Iy,Iz, c, RBF_Means, RBF_Stds, W, u1_prev, u2_prev, u3_prev, u4_prev)

%g = 9.81;
%mass = 1; L = 0.6; 
%Ix = 0.85; 
%Iy = 0.85; 
%Iz = Ix+Iy;
%c = 0.088; 
phiddes = 0;
phidddes = 0;

%thetades = 0.0*pi/180;
thetaddes = 0;
thetadddes = 0;
%phides = 0.0*pi/180;

%xdes = 0;
xddes = 0;
xdddes = 0;
%ydes = 0;
yddes = 0;
ydddes = 0;
%zdes = 0;
zddes = 0;
zdddes = 0;
%psides = 0*pi/180;
psiddes = 0;
psidddes = 0;

%phides=0;
%thetades=0;
%if zdes<0
%zdes=0.5;
%end

%% NN
% neural net inputs
Gamma = 100;
e_z = z - zdes;
e_dot_z = zd - zddes;
x_n = [phi/10; theta/10; psi/10; z/10; zdes/15];
x_dot_n = [phid/10; thetad/10; psid/10; zd/10; e_dot_z*2];
u = [u2_prev; u3_prev; u4_prev; u1_prev];
u_n = u/15;
nn_input = [x_n; x_dot_n; u_n];

% e_n = z - zdes;
% e_dot_n = zd - zddes;
% x_n = z;
% x_dot_n = zd;
% u = u1_prev;
% u_n = u;
% nn_input = [x_n/10; x_dot_n/10; e_n; e_dot_n*2; u_n/15];


mu = zeros(40, 1);
for i = 1 : 40
    mu(i, 1) = exp(-norm(nn_input - RBF_Means(:, i))^2/(2 * RBF_Stds(i)^2));
end

% estimation of uncertainties
Delta_hat = transpose(W) * mu;


%% Back stepping
% cz = 10; ghat = 1 * g; eta1 = 50;
% s1 = cz*(z - zdes) + (zd - zddes);
% u1 = (mass/(cos(phi)*cos(theta)))*(cz*(zd-zddes) - zdddes + ghat + eta1*s1 + Delta_hat);

%%
ghat = 1 * g; cz = 1; masshat = mass;
eps1 = 0.8;
eta1 = 50;
s1 = cz*(z - zdes) + 1*(zd - zddes);
% if s1 > 1
%     sgn1 = 1;
% elseif   s1 < -1
%     sgn1 = -1;
% else
%     sgn1 = s1;
% end
sgn1 = tanh(s1);
u1_nn = (masshat/(cos(phi)*cos(theta)))*(cz*(zd-(zddes)) + zdddes + ghat + eps1*sgn1 + eta1*s1 + Delta_hat(4));
u1 = (masshat/(cos(phi)*cos(theta)))*(cz*(zd-(zddes)) + zdddes + ghat + eps1*sgn1 + eta1*s1);
%%
cpsi = 1.5; eps2 = 0.8; eta2 = 50; 
Izhat = 1 * Iz; chat = 1 * c;
s2 = cpsi*(psides - psi) + (psiddes - psid);
% if s2 > 1
%     sgn2 = 1;
% elseif   s2 < -1
%     sgn2 = -1;
% else
%     sgn2 = s2;
% end
sgn2 = tanh(s2);
u4_nn = (Izhat/chat)*(cpsi*(psiddes-psid) + psidddes + eps2*sgn2 + eta2*s2 + 0.43*Delta_hat(3));
u4 = (Izhat/chat)*(cpsi*(psiddes-psid) + psidddes + eps2*sgn2 + eta2*s2);
%% 
eps3 = 0.5; eta3 = 50; ctheta = 1.5;
Iyhat = 1 * Iy; Ixhat = 1 * Ix; lhat = 1 * L;
c3 = 0.5;
% c1 = (11*mass/(u1*cos(phi)*cos(psi)*cos(thetades))) * c3;
% c2 = (6*mass/(u1*cos(phi)*cos(psi)*cos(thetades))) * c3;
c1 = (11*mass/(cos(phi)*cos(psi)*cos(thetades))) * c3;
c2 = (6*mass/(cos(phi)*cos(psi)*cos(thetades))) * c3;
% c4 = (6) * c3;
c4 = 0.5;
s3 = c1*(xddes - xd) + c2*(xdes - x) + c3*(thetaddes - thetad) + c4*(thetades - theta);
% s5 = 0.1*(xddes - xd) + 0.10*(xdes - x);
% s3 = c3*(thetaddes - thetad) + c4*(thetades- theta);

% if s3 > 1
%     sgn3 = 1;
% elseif   s3 < -1
%     sgn3 = -1;
% else
%     sgn3 = s3;
% end
sgn3 = tanh(s3);
u3_nn = (Iyhat/lhat)*((c1/c3)*(xdddes-xdd) + (c2/c3)*(xddes-xd) + thetadddes ...
       + (c4/c3)*(thetaddes-thetad)  + (1/c3)*(eps3*sgn3 + eta3*s3) + Delta_hat(2));

u3 = (Iyhat/lhat)*((c1/c3)*(xdddes-xdd) + (c2/c3)*(xddes-xd) + thetadddes ...
       + (c4/c3)*(thetaddes-thetad)  + (1/c3)*(eps3*sgn3 + eta3*s3));

% u3 = (Iyhat/chat)*(ctheta*(thetaddes-thetad) + thetadddes + eps3*sgn3 + eta3*s3);

%u3(st) = 0;
%%
eps4 = 0.5; eta4 = 50; chphi = 1.5;
% c7 = 1;
c7 = 0.5;
% c5 = (-11*mass/((u1*sin(phides)*sin(theta)*sin(psi))+(u1*cos(phides)*cos(psi)))) * c7;
% c6 = (-6*mass/((u1*sin(phides)*sin(theta)*sin(psi))+(u1*cos(phides)*cos(psi)))) * c7;
% c5 = (-11*mass/((sin(phides)*sin(theta)*sin(psi))+(u1*cos(phides)*cos(psi)))) * c7;
% c6 = (-6*mass/((sin(phides)*sin(theta)*sin(psi))+(u1*cos(phides)*cos(psi)))) * c7;
c5 = (-11*mass/((sin(phides)*sin(theta)*sin(psi))+(cos(phides)*cos(psi)))) * c7;
c6 = (-6*mass/((sin(phides)*sin(theta)*sin(psi))+(cos(phides)*cos(psi)))) * c7;
c8 = 0.5;

s4 = c5*(yddes - yd) + c6*(ydes - y) + c7*(phiddes - phid) + c8*(phides - phi);
s6 = -0.1*(yddes - yd) + -0.1*(ydes - y);
% s4 = c7*(phiddes - phid) + c8*(phides - phi);
% if s4 > 1
%     sgn4 = 1;
% elseif   s4 < -1
%     sgn4 = -1;
% else
%     sgn4 = s4;
% end
sgn4 = tanh(s4);
u2_nn = (Ixhat/lhat)*((c5/c7)*(ydddes-ydd) + (c6/c7)*(yddes-yd) + phidddes ...
        + (c8/c7)*(phiddes-phid) +  (1/c7)*(eps4*sgn4 + eta4*s4) + Delta_hat(1));

u2 = (Ixhat/lhat)*((c5/c7)*(ydddes-ydd) + (c6/c7)*(yddes-yd) + phidddes ...
        + (c8/c7)*(phiddes-phid) +  (1/c7)*(eps4*sgn4 + eta4*s4));

% u2 = (Ixhat/lhat)*(chphi*(phiddes-phid) + phidddes + eps4*sgn4 + eta4*s4);

s = [s4; s3; s2; s1];
% s = s1;
W_dot = Gamma * mu * s';

== matlab function Altitude_SMCIBVS_RBFSMC/Neuro-adaptive Sliding Mode Control/Subsystem/MATLAB Function1 ==
  data: u input; y output
function y = fcn(u)

y = u;

== matlab function Altitude_SMCIBVS_RBFSMC/Neuro-adaptive Sliding Mode Control/Subsystem/MATLAB Function2 ==
  data: u input; y output
function y = fcn(u)

y = u;

== matlab function Altitude_SMCIBVS_RBFSMC/Image-based Visual Servo/Image-based Visual Servo ==
  data: t input; reference input; projection input; u_inertial output; u output; phi_ang input; theta input; psi input; phi_bound input; d_error input; error output; v_features output; u_prev_out output; u_prev_in input; SSE output; d_hat_out output; d_hat_prev input; Kp_prev output; Kd_prev output; Kq_prev output; Kp input; Kd input; Kq input
function [u_inertial, u, error, v_features, u_prev_out, SSE, d_hat_out, Kp_prev, Kd_prev, Kq_prev]   = compute_control_inputs(t, reference, projection, phi_ang, theta, psi, phi_bound, d_error, u_prev_in, d_hat_prev, Kp, Kd, Kq)


x_i1 = projection(1);         % x projection in the image plane
y_i1 = projection(2);         % y projection
z_c1 = projection(3);
x_i2 = projection(4);
y_i2 = projection(5);
z_c2 = projection(6);
x_i3 = projection(7);         % x projection in the image plane
y_i3 = projection(8);         % y projection
z_c3 = projection(9);
x_i4 = projection(10);
y_i4 = projection(11);
z_c4 = projection(12);

% It's CRITICAL that z_c values are never zero.
% if z_c1 == 0, z_c1 = 1e-3; end % Avoid division by zero
% if z_c2 == 0, z_c2 = 1e-3; end
% if z_c3 == 0, z_c3 = 1e-3; end
% if z_c4 == 0, z_c4 = 1e-3; end

projection_vec = [x_i1; y_i1; x_i2; y_i2; x_i3; y_i3; x_i4; y_i4];
error = reference - projection_vec;

SSE = error' * error;   


Ls1 = [ -1/z_c1     0     x_i1/z_c1     x_i1*y_i1    -(1+x_i1^2)     y_i1;  
        0       -1/z_c1   y_i1/z_c1    1+y_i1^2      -x_i1*y_i1     -x_i1];
    
Ls2 = [ -1/z_c2     0     x_i2/z_c2     x_i2*y_i2    -(1+x_i2^2)     y_i2;  
        0       -1/z_c2   y_i2/z_c2    1+y_i2^2      -x_i2*y_i2     -x_i2];
Ls3 = [ -1/z_c3     0     x_i3/z_c3     x_i3*y_i3    -(1+x_i3^2)     y_i3;  
        0       -1/z_c3   y_i3/z_c3    1+y_i3^2      -x_i3*y_i3     -x_i3];
    
Ls4 = [ -1/z_c4     0     x_i4/z_c4     x_i4*y_i4    -(1+x_i4^2)     y_i4;  
        0       -1/z_c4   y_i4/z_c4    1+y_i4^2      -x_i4*y_i4     -x_i4];
    
Ls = [Ls1; Ls2; Ls3; Ls4]; 


% Kd = diag([0.05, 0.05, 0.05, 0.05, 0.05, 0.05, 0.05, 0.05])*150; 
% Kp = diag([6, 6, 6, 6, 6, 6, 6, 6])*2.5;
% Kq = diag([0.01, 0.01, 0.01, 0.01, 0.01, 0.01, 0.01, 0.01])*80;

tanh_term = tanh(error / phi_bound); 

%%
tau = 0.6;                 % 0 < tau < 1   (smoothing factor)
compensation_factor = 0.5; % partial compensation

% everything except proportional part
dist_signal = Kd * d_error + Kq * tanh_term;

% first-order low-pass estimate of disturbance
d_hat = (1 - tau) * d_hat_prev + tau * dist_signal;

% control features with partial disturbance compensation
v_features = Kp * error + dist_signal - compensation_factor * d_hat;

% output state for next step
d_hat_out = d_hat;

%%


% v_features = Kp * error + Kd * d_error + Kq * tanh_term;
v_features = Kp * error + Kq * tanh_term;

u = pinv(Ls) * v_features; 


% Rotation matrix (Inertial to Body)
Rx = [1 0 0; 0 cos(phi_ang) sin(phi_ang); 0 -sin(phi_ang) cos(phi_ang)];
Ry = [cos(theta) 0 -sin(theta); 0 1 0; sin(theta) 0 cos(theta)];
Rz = [cos(psi) sin(psi) 0; -sin(psi) cos(psi) 0; 0 0 1];
R = Rx * Ry * Rz; 

% Transformation matrix (Body to Inertial angular rates)
J2 = [1 sin(phi_ang)*tan(theta) cos(phi_ang)*tan(theta); 
      0 cos(phi_ang) -sin(phi_ang); 
      0 sin(phi_ang)/cos(theta) cos(phi_ang)/cos(theta)];


v_body = u(1:3);
w_body = u(4:6);

v_inertial = R' * v_body;      % R' is R_body_to_inertial
w_inertial = J2 * w_body;      % J2 is R_body_to_inertial_rates

u_inertial = [v_inertial; w_inertial];

beta = 0.8;
% u_inertial = beta * u_prev_in + (1 - beta) * u_inertial;
u_prev_out = u_inertial;

Kd_prev = Kd;
Kp_prev = Kp;
Kq_prev = Kq;

end

== matlab function Altitude_SMCIBVS_RBFSMC/Image-based Visual Servo/MATLAB Function5 ==
  data: u1 input; y output; u2 input; dt input
function y = fcn(u1,u2,dt)

y = (u2-u1)/dt;

== matlab function Altitude_SMCIBVS_RBFSMC/Image-based Visual Servo/Gain Optimizer/MATLAB Function ==
  data: u input; y output
function y = fcn(u)
m=length(u);
y=0;
for i=1:m
    y=y+(u(i)^2);
end
y = y^0.5;

== matlab function Altitude_SMCIBVS_RBFSMC/Quad Dynamic Model/Quadrotor Dynamic Model ==
  data: t input; u1 input; u2 input; u3 input; u4 input; p input; pdot output; q input; r input; qdot output; rdot output; phi input; theta input; psi input; u input; v input; w input; xd input; yd input; zd input; phid output; thetad output; psid output; udot output; vdot output; wdot output; xdd output; ydd output; zdd output; g input; mass input; L input; Ixx input; Iyy input; Izz input; Delta output
function [pdot, qdot, rdot, phid, thetad, psid, udot, vdot, wdot, xdd, ydd, zdd, Delta] = fcn(t, u1, u2, u3, u4, p, q, r, phi, theta, psi, u, v, w, xd, yd, zd, g, mass, L, Ixx, Iyy, Izz)


% k1 = 0.1; k2 = 0.1; k3 = 0.1; k4 = 0.12; k5 = 0.12; k6 = 0.12;
 
%Izz = Ixx+Iyy;

phid = p + q*sin(phi)*tan(theta) + r*cos(phi)*tan(theta);
thetad = q*cos(phi) - r*sin(phi);
psid = q*sin(phi)*sec(theta) + r*cos(phi)*sec(theta);

Delta1 = [phi * theta; theta * psi; phi * psi; 0.2 * zd];
d1 = [10*0.5 * sin(pi * t/2); 10*0.5 * sin(pi * t/3); 10*0.2 * sin(pi * t); 6*sin(2 * pi * t + pi/6)];
Delta = Delta1 + d1;

pdot = r*q*(Iyy - Izz)/Ixx + (u2)/Ixx - Delta(1);
qdot = r*p*(Izz - Ixx)/Iyy + (u3)/Iyy - Delta(2);
rdot = p*q*(Ixx - Iyy)/Izz + (u4)/Izz - Delta(3);


udot = r*v - q*w -g*sin(theta);
vdot = p*w - u*r +g*cos(theta)*sin(phi); 
wdot = q*u - p*v +g*cos(theta)*cos(phi) - u1/mass;

% AA = [cos(psi)*cos(theta), -sin(psi)*cos(phi)+cos(psi)*sin(theta)*sin(phi), sin(psi)*sin(phi)+cos(psi)*sin(theta)*cos(phi);
%      sin(psi)*cos(theta), cos(psi)*cos(phi)+sin(psi)*sin(theta)*sin(phi), -sin(phi)*cos(psi)+sin(psi)*sin(theta)*cos(phi);
%     -sin(theta), cos(theta)*sin(phi), cos(theta)*cos(phi)]; 
% 
% xd = AA(1,:)*[u;v;w];
% yd = AA(2,:)*[u;v;w];
% zd = AA(3,:)*[u;v;w];

% xdd = (-u1/mass)*(sin(phi)*sin(psi)+cos(phi)*cos(psi)*sin(theta));
% ydd = (-u1/mass)*(cos(phi)*sin(psi)*sin(theta)-cos(psi)*sin(phi));
% zdd = g + (-u1/mass)*(cos(phi)*cos(theta));

xdd = (1/mass)*(cos(phi)*sin(theta)*cos(psi)+sin(phi)*sin(psi))*u1 ;
ydd = (1/mass)*(sin(psi)*sin(theta)*cos(phi)-cos(psi)*sin(phi))*u1 ;
zdd = -(1/mass)*(cos(phi)*cos(theta))*u1+g + Delta(4);
